simulink model "closedLoop"  (R2021b)
settings: Solver=FixedStepAuto  StartTime=0.0  StopTime=inf  FixedStep=0.001  RelTol=1e-3
settings Model: Creator=marko  LastModifiedBy=marko

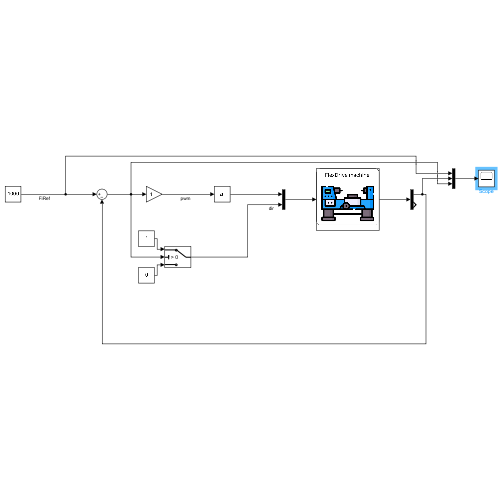
[thumbnail: Simulink's stored preview of the top-level diagram]
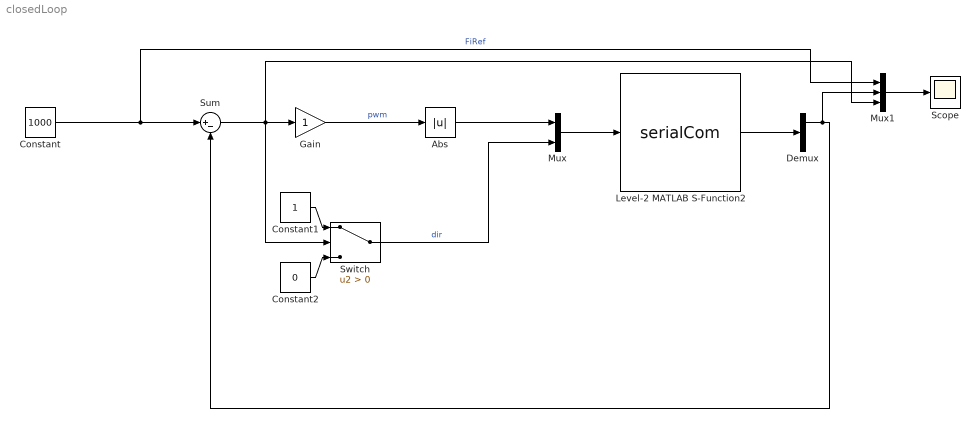
== system closedLoop ==
  Abs : Abs
  Constant : Constant  Value=1000
  Constant1 : Constant
  Constant2 : Constant  Value=0
  Demux : Demux  Outputs=2
  Gain : Gain
  Level-2 MATLAB S-Function2 : M-S-Function  FunctionName=serialCom  Parameters='COM9', 115200
      mask Display: image('$imagefile'); % Use "Edit Image" on toolstrip to change.
  Mux : Mux  Inputs=2
  Mux1 : Mux  Inputs=3
  Scope : Scope
  Sum : Sum  Inputs=|+-
  Switch : Switch  Criteria=u2 > Threshold
  wires:
  Level-2 MATLAB S-Function2/1 -> Demux/1
  Mux/1 -> Level-2 MATLAB S-Function2/1
  Constant/1 -> Mux1/1, Sum/1  "FiRef"
  Sum/1 -> Mux1/3, Switch/2, Gain/1
  Demux/1 -> Mux1/2, Sum/2
  Gain/1 -> Abs/1  "pwm"
  Switch/1 -> Mux/2  "dir"
  Constant1/1 -> Switch/1
  Constant2/1 -> Switch/3
  Mux1/1 -> Scope/1
  Abs/1 -> Mux/1
